simulink model "Filter_attivo"  (R2016b)
settings: Solver=ode23t  StartTime=0.0  StopTime=2.4  MaxStep=1e-4  RelTol=1e-3  EnableMultiTasking=on
values from neighbouring files (symbols this model uses):
  ampiezza_rete = 150/sqrt(3)    [Data.m]    (also in taratura.m)
  C = 2.2e-3    (= 0.0022)    [Data.m]
  C_raddr = 600e-6    (= 0.0006)    [Data.m]
  f = 50    [Data.m]    (also in Spettro_complesso.m = bar(-fp((26:25:25000-25)),PyTHD(length(PyTHD)-1:-1:length(Py)
  f_am = 500    [Data.m]
  h = Lagrange_coef(f,1/Tc)    [Data.m]    (also in Lagrange_coef.m = NaN(4,round(fc/f1*0.5)))
  h_rit = Lagrange_coef_rit(1.5)    [Data.m]
  k_interno = 0.99    [tuning.m]
  k_par_AM = 10    [Data.m]
  ki_PI = 0.2    [Data.m]
  ki_PLL = 1000    [Data.m]
  ki_ris = 47.5*2    (= 95)    [Data.m]
  kp_PI = 1.57    [Data.m]
  kp_PLL = 0.9    [Data.m]
  kp_ris = 47.5*0.089*2    (= 8.455)    [Data.m]
  L_disaccoppiamento = 2*1.18e-3    (= 0.00236)    [Data.m]    (also in taratura.m)
  L_rete = 4e-3    (= 0.004)    [Data.m]    (also in tuning.m)
  max_PI = 8    [Data.m]
  max_PLL = 1000    [Data.m]
  min_PI = -8    [Data.m]
  min_PLL = -1000    [Data.m]
  Notch_z = 1-Peaking_z    [Data.m]
  Notch_z_AM1 = 1-Peaking_z_AM1    [Notch.m]
  peak_rete = Peaking(f,1/Tc,0.1)    [Data.m]
  Peaking_dir1_d = c2d(Peaking_dir1_s,1/fs,'tustin')    [semipeaking.m]
  pendenza = 1000    [Data.m]
  R_carico = 50    [Data.m]
  R_disaccoppiamento = 2*13e-3    (= 0.026)    [Data.m]    (also in taratura.m)
  R_raddr = 60    [Data.m]
  R_rete = 100e-3    (= 0.1)    [Data.m]    (also in tuning.m = 0.01)
  T = 20e-3    (= 0.02)    [Data.m]    (also in tuning.m)
  tau_filtro_Vdc_ref = 0.15    [Data.m]
  Tc = 1/10000    (= 0.0001)    [Data.m]    (also in taratura.m; tuning.m)
  Vdc_ref = 200    [Data.m]    (also in taratura.m)
  w_filtro = 2*pi*f_taglio    (= 56548.6677646)    [Data.m]
undefined symbols (not defined in the file or in its folder): DiscIntNeverNeededParam, k_par, k_ser, Notch_z_AM1_5, Notch_z_AM1_7, Notch_z_AM2_5, Notch_z_AM2_7, Peaking_inv_d, plecs, Q_inv
libraries: powerlib x54, simulink x8, powerlib_extras x4, powerlib_meascontrol x2
(part 5 of 5)

== system Filter_attivo/Controllo tensione/Controllo ripetitivo/Controllo ripetitivo/Regolatore ripetitivo/vecchi controlli/Ripetitivo Modulazione AM1/Banco di ripetitivi/rep_comp 5 ==
  In1 : Inport
  Add1 : Sum  Inputs=-+
  Delay1 : Delay
  Delay3 : Delay  DelayLength=fix(1/(Tc*f*1*ro)-1-rit)
  Discrete FIR Filter : DiscreteFir  Coefficients=[h(1,ro) h(2,ro) h(3,ro) h(4,ro)]
  Gain : Gain  Gain=0.98
  Gain1 : Gain  Gain=g_interno
  Scope2 : Subsystem  LoadFcn=plecs('sl', 300);  InitFcn=plecs('sl', 314);  StartFcn=plecs('sl', 308);  StopFcn=plecs('sl', 309);  mask{Settings=<binary blob, 216 chars, not shown>}
      mask init:
      | plecs('sl', 315);
      settings: CopyFcn=plecs('sl', 303);  DeleteFcn=plecs('sl', 305);  UndoDeleteFcn=plecs('sl', 306);  PreSaveFcn=plecs('sl', 311);  NameChangeFcn=plecs('sl', 310);  DestroyFcn=plecs('sl', 307);  OpenFcn=plecs('sl', 302);  ErrorFcn=plerrorfcn
      mask Display: plot([0.1 0.9 0.9 0.1 0.1], [0.9 0.9 0.5 0.5 0.9])
  Out1 : Outport
  wires:
  Gain1/1 -> Out1/1, Scope2/1(1)
  Discrete FIR Filter/1 -> Gain/1, Gain1/1
  Gain/1 -> Delay1/1
  Delay1/1 -> Add1/2
  Add1/1 -> Delay3/1
  In1/1 -> Add1/1
  Delay3/1 -> Discrete FIR Filter/1

== system Filter_attivo/Controllo tensione/Controllo ripetitivo/Controllo ripetitivo/Regolatore ripetitivo/vecchi controlli/Ripetitivo Modulazione AM1/Banco di ripetitivi/rep_comp 6 ==
  In1 : Inport
  Add1 : Sum  Inputs=-+
  Delay1 : Delay
  Delay3 : Delay  DelayLength=fix(1/(Tc*f*1*ro)-1-rit)
  Discrete FIR Filter : DiscreteFir  Coefficients=[h(1,ro) h(2,ro) h(3,ro) h(4,ro)]
  Gain : Gain  Gain=0.98
  Gain1 : Gain  Gain=g_interno
  Scope2 : Subsystem  LoadFcn=plecs('sl', 300);  InitFcn=plecs('sl', 314);  StartFcn=plecs('sl', 308);  StopFcn=plecs('sl', 309);  mask{Settings=<binary blob, 216 chars, not shown>}
      mask init:
      | plecs('sl', 315);
      settings: CopyFcn=plecs('sl', 303);  DeleteFcn=plecs('sl', 305);  UndoDeleteFcn=plecs('sl', 306);  PreSaveFcn=plecs('sl', 311);  NameChangeFcn=plecs('sl', 310);  DestroyFcn=plecs('sl', 307);  OpenFcn=plecs('sl', 302);  ErrorFcn=plerrorfcn
      mask Display: plot([0.1 0.9 0.9 0.1 0.1], [0.9 0.9 0.5 0.5 0.9])
  Out1 : Outport
  wires:
  Delay3/1 -> Discrete FIR Filter/1
  In1/1 -> Add1/1
  Add1/1 -> Delay3/1
  Delay1/1 -> Add1/2
  Gain/1 -> Delay1/1
  Discrete FIR Filter/1 -> Gain1/1, Gain/1
  Gain1/1 -> Scope2/1(1), Out1/1

== system Filter_attivo/Controllo tensione/Controllo ripetitivo/Controllo ripetitivo/Regolatore ripetitivo/vecchi controlli/Ripetitivo Modulazione AM1/Banco notch 5_7_AM/notch_demodulazione_5_1 ==
  In1 : Inport
  Discrete Transfer Fcn : DiscreteTransferFcn  Numerator=cell2mat(Notch_z_AM1_5.num)  Denominator=cell2mat(Notch_z_AM1_5.den)
  Discrete Transfer Fcn1 : DiscreteTransferFcn  Numerator=cell2mat(Notch_z_AM2_5.num)  Denominator=cell2mat(Notch_z_AM2_5.den)
  Discrete Transfer Fcn2 : DiscreteTransferFcn  Numerator=cell2mat(Notch_z_AM1_7.num)  Denominator=cell2mat(Notch_z_AM1_7.den)
  Discrete Transfer Fcn3 : DiscreteTransferFcn  Numerator=cell2mat(Notch_z_AM2_7.num)  Denominator=cell2mat(Notch_z_AM2_7.den)
  Out1 : Outport
  wires:
  Discrete Transfer Fcn2/1 -> Out1/1
  In1/1 -> Discrete Transfer Fcn/1
  Discrete Transfer Fcn/1 -> Discrete Transfer Fcn1/1
  Discrete Transfer Fcn1/1 -> Discrete Transfer Fcn3/1
  Discrete Transfer Fcn3/1 -> Discrete Transfer Fcn2/1

== system Filter_attivo/Controllo tensione/Controllo ripetitivo/Controllo ripetitivo/Regolatore ripetitivo/vecchi controlli/Ripetitivo Modulazione AM1/Banco notch 5_7_AM/notch_demodulazione_5_7 ==
  In1 : Inport
  Discrete Transfer Fcn : DiscreteTransferFcn  Numerator=cell2mat(Notch_z_AM1_5.num)  Denominator=cell2mat(Notch_z_AM1_5.den)
  Discrete Transfer Fcn1 : DiscreteTransferFcn  Numerator=cell2mat(Notch_z_AM2_5.num)  Denominator=cell2mat(Notch_z_AM2_5.den)
  Discrete Transfer Fcn2 : DiscreteTransferFcn  Numerator=cell2mat(Notch_z_AM1_7.num)  Denominator=cell2mat(Notch_z_AM1_7.den)
  Discrete Transfer Fcn3 : DiscreteTransferFcn  Numerator=cell2mat(Notch_z_AM2_7.num)  Denominator=cell2mat(Notch_z_AM2_7.den)
  Out1 : Outport
  wires:
  Discrete Transfer Fcn3/1 -> Discrete Transfer Fcn2/1
  Discrete Transfer Fcn1/1 -> Discrete Transfer Fcn3/1
  Discrete Transfer Fcn/1 -> Discrete Transfer Fcn1/1
  In1/1 -> Discrete Transfer Fcn/1
  Discrete Transfer Fcn2/1 -> Out1/1

== system Filter_attivo/Controllo tensione/Controllo ripetitivo/Controllo ripetitivo/Regolatore ripetitivo/vecchi controlli/Ripetitivo Modulazione AM1/Scope1/ InputMux  ==
  In1 : Inport
  Convert1 : DataTypeConversion  SaturateOnIntegerOverflow=on  RndMeth=Zero
  Mux : Mux  Inputs=1
  Out : Outport
  wires:
  Mux/1 -> Out/1
  In1/1 -> Convert1/1
  Convert1/1 -> Mux/1

== system Filter_attivo/Controllo tensione/Controllo ripetitivo/Controllo ripetitivo/Regolatore ripetitivo/Ripetitivo Modulazione AM/Banco di ripetitivi/rep_comp 1/Scope2/ InputMux  ==
  In1 : Inport
  Convert1 : DataTypeConversion  SaturateOnIntegerOverflow=on  RndMeth=Zero
  Mux : Mux  Inputs=1
  Out : Outport
  wires:
  Mux/1 -> Out/1
  In1/1 -> Convert1/1
  Convert1/1 -> Mux/1

== system Filter_attivo/Controllo tensione/Controllo ripetitivo/Controllo ripetitivo/Regolatore ripetitivo/Ripetitivo Modulazione AM/Banco di ripetitivi/rep_comp 2/Scope2/ InputMux  ==
  In1 : Inport
  Convert1 : DataTypeConversion  SaturateOnIntegerOverflow=on  RndMeth=Zero
  Mux : Mux  Inputs=1
  Out : Outport
  wires:
  Convert1/1 -> Mux/1
  In1/1 -> Convert1/1
  Mux/1 -> Out/1

== system Filter_attivo/Controllo tensione/Controllo ripetitivo/Controllo ripetitivo/Regolatore ripetitivo/Ripetitivo Modulazione AM/Banco di ripetitivi/rep_comp 3/Scope2/ InputMux  ==
  In1 : Inport
  Convert1 : DataTypeConversion  SaturateOnIntegerOverflow=on  RndMeth=Zero
  Mux : Mux  Inputs=1
  Out : Outport
  wires:
  Mux/1 -> Out/1
  In1/1 -> Convert1/1
  Convert1/1 -> Mux/1

== system Filter_attivo/Controllo tensione/Controllo ripetitivo/Controllo ripetitivo/Regolatore ripetitivo/Ripetitivo Modulazione AM/Banco di ripetitivi/rep_comp 4/Scope2/ InputMux  ==
  In1 : Inport
  Convert1 : DataTypeConversion  SaturateOnIntegerOverflow=on  RndMeth=Zero
  Mux : Mux  Inputs=1
  Out : Outport
  wires:
  Convert1/1 -> Mux/1
  In1/1 -> Convert1/1
  Mux/1 -> Out/1

== system Filter_attivo/Controllo tensione/Controllo ripetitivo/Controllo ripetitivo/Regolatore ripetitivo/Ripetitivo Modulazione AM/Banco di ripetitivi/rep_comp 5/Scope2/ InputMux  ==
  In1 : Inport
  Convert1 : DataTypeConversion  SaturateOnIntegerOverflow=on  RndMeth=Zero
  Mux : Mux  Inputs=1
  Out : Outport
  wires:
  Mux/1 -> Out/1
  In1/1 -> Convert1/1
  Convert1/1 -> Mux/1

== system Filter_attivo/Controllo tensione/Controllo ripetitivo/Controllo ripetitivo/Regolatore ripetitivo/Ripetitivo Modulazione AM/Banco di ripetitivi/rep_comp 6/Scope2/ InputMux  ==
  In1 : Inport
  Convert1 : DataTypeConversion  SaturateOnIntegerOverflow=on  RndMeth=Zero
  Mux : Mux  Inputs=1
  Out : Outport
  wires:
  Convert1/1 -> Mux/1
  In1/1 -> Convert1/1
  Mux/1 -> Out/1

== system Filter_attivo/Controllo tensione/Controllo ripetitivo/Controllo ripetitivo/Regolatore ripetitivo/vecchi controlli/Ripetitivo Modulazione AM1/Banco di ripetitivi/rep_comp 1/Scope2 ==
  1 : Inport
  " InputMux " : Subsystem
      mask Display: disp('Mux')
  " S-Function " : S-Function  FunctionName=plecs  SFunctionDeploymentMode=off  EnableBusSupport=off
  wires:
  1/1 -> " InputMux "/1(In1)
  " InputMux "/1(Out) -> " S-Function "/1

== system Filter_attivo/Controllo tensione/Controllo ripetitivo/Controllo ripetitivo/Regolatore ripetitivo/vecchi controlli/Ripetitivo Modulazione AM1/Banco di ripetitivi/rep_comp 2/Scope2 ==
  1 : Inport
  " InputMux " : Subsystem
      mask Display: disp('Mux')
  " S-Function " : S-Function  FunctionName=plecs  SFunctionDeploymentMode=off  EnableBusSupport=off
  wires:
  " InputMux "/1(Out) -> " S-Function "/1
  1/1 -> " InputMux "/1(In1)

== system Filter_attivo/Controllo tensione/Controllo ripetitivo/Controllo ripetitivo/Regolatore ripetitivo/vecchi controlli/Ripetitivo Modulazione AM1/Banco di ripetitivi/rep_comp 3/Scope2 ==
  1 : Inport
  " InputMux " : Subsystem
      mask Display: disp('Mux')
  " S-Function " : S-Function  FunctionName=plecs  SFunctionDeploymentMode=off  EnableBusSupport=off
  wires:
  1/1 -> " InputMux "/1(In1)
  " InputMux "/1(Out) -> " S-Function "/1

== system Filter_attivo/Controllo tensione/Controllo ripetitivo/Controllo ripetitivo/Regolatore ripetitivo/vecchi controlli/Ripetitivo Modulazione AM1/Banco di ripetitivi/rep_comp 4/Scope2 ==
  1 : Inport
  " InputMux " : Subsystem
      mask Display: disp('Mux')
  " S-Function " : S-Function  FunctionName=plecs  SFunctionDeploymentMode=off  EnableBusSupport=off
  wires:
  " InputMux "/1(Out) -> " S-Function "/1
  1/1 -> " InputMux "/1(In1)

== system Filter_attivo/Controllo tensione/Controllo ripetitivo/Controllo ripetitivo/Regolatore ripetitivo/vecchi controlli/Ripetitivo Modulazione AM1/Banco di ripetitivi/rep_comp 5/Scope2 ==
  1 : Inport
  " InputMux " : Subsystem
      mask Display: disp('Mux')
  " S-Function " : S-Function  FunctionName=plecs  SFunctionDeploymentMode=off  EnableBusSupport=off
  wires:
  1/1 -> " InputMux "/1(In1)
  " InputMux "/1(Out) -> " S-Function "/1

== system Filter_attivo/Controllo tensione/Controllo ripetitivo/Controllo ripetitivo/Regolatore ripetitivo/vecchi controlli/Ripetitivo Modulazione AM1/Banco di ripetitivi/rep_comp 6/Scope2 ==
  1 : Inport
  " InputMux " : Subsystem
      mask Display: disp('Mux')
  " S-Function " : S-Function  FunctionName=plecs  SFunctionDeploymentMode=off  EnableBusSupport=off
  wires:
  " InputMux "/1(Out) -> " S-Function "/1
  1/1 -> " InputMux "/1(In1)

== system Filter_attivo/Controllo tensione/Controllo ripetitivo/Controllo ripetitivo/Regolatore ripetitivo/vecchi controlli/Ripetitivo Modulazione AM1/Banco di ripetitivi/rep_comp 1/Scope2/ InputMux  ==
  In1 : Inport
  Convert1 : DataTypeConversion  SaturateOnIntegerOverflow=on  RndMeth=Zero
  Mux : Mux  Inputs=1
  Out : Outport
  wires:
  Convert1/1 -> Mux/1
  In1/1 -> Convert1/1
  Mux/1 -> Out/1

== system Filter_attivo/Controllo tensione/Controllo ripetitivo/Controllo ripetitivo/Regolatore ripetitivo/vecchi controlli/Ripetitivo Modulazione AM1/Banco di ripetitivi/rep_comp 2/Scope2/ InputMux  ==
  In1 : Inport
  Convert1 : DataTypeConversion  SaturateOnIntegerOverflow=on  RndMeth=Zero
  Mux : Mux  Inputs=1
  Out : Outport
  wires:
  Mux/1 -> Out/1
  In1/1 -> Convert1/1
  Convert1/1 -> Mux/1

== system Filter_attivo/Controllo tensione/Controllo ripetitivo/Controllo ripetitivo/Regolatore ripetitivo/vecchi controlli/Ripetitivo Modulazione AM1/Banco di ripetitivi/rep_comp 3/Scope2/ InputMux  ==
  In1 : Inport
  Convert1 : DataTypeConversion  SaturateOnIntegerOverflow=on  RndMeth=Zero
  Mux : Mux  Inputs=1
  Out : Outport
  wires:
  Convert1/1 -> Mux/1
  In1/1 -> Convert1/1
  Mux/1 -> Out/1

== system Filter_attivo/Controllo tensione/Controllo ripetitivo/Controllo ripetitivo/Regolatore ripetitivo/vecchi controlli/Ripetitivo Modulazione AM1/Banco di ripetitivi/rep_comp 4/Scope2/ InputMux  ==
  In1 : Inport
  Convert1 : DataTypeConversion  SaturateOnIntegerOverflow=on  RndMeth=Zero
  Mux : Mux  Inputs=1
  Out : Outport
  wires:
  Mux/1 -> Out/1
  In1/1 -> Convert1/1
  Convert1/1 -> Mux/1

== system Filter_attivo/Controllo tensione/Controllo ripetitivo/Controllo ripetitivo/Regolatore ripetitivo/vecchi controlli/Ripetitivo Modulazione AM1/Banco di ripetitivi/rep_comp 5/Scope2/ InputMux  ==
  In1 : Inport
  Convert1 : DataTypeConversion  SaturateOnIntegerOverflow=on  RndMeth=Zero
  Mux : Mux  Inputs=1
  Out : Outport
  wires:
  Convert1/1 -> Mux/1
  In1/1 -> Convert1/1
  Mux/1 -> Out/1

== system Filter_attivo/Controllo tensione/Controllo ripetitivo/Controllo ripetitivo/Regolatore ripetitivo/vecchi controlli/Ripetitivo Modulazione AM1/Banco di ripetitivi/rep_comp 6/Scope2/ InputMux  ==
  In1 : Inport
  Convert1 : DataTypeConversion  SaturateOnIntegerOverflow=on  RndMeth=Zero
  Mux : Mux  Inputs=1
  Out : Outport
  wires:
  Mux/1 -> Out/1
  In1/1 -> Convert1/1
  Convert1/1 -> Mux/1

== matlab function Filter_attivo/Rete/generatore diretta e inversa/MATLAB Function ==
  data: teta input; v_a output; a_d input; a_i input; v_b output; v_c output; fase_i input
function [v_a,v_b,v_c] = fcn(teta,a_d,a_i,fase_i)

alfa=exp(2/3*pi*1i);
alfa_q=exp(-2/3*pi*1i);
vd_c=a_d*exp(-teta*1i);
v1_d=real(vd_c);
v2_d=real(vd_c*alfa_q);
v3_d=real(vd_c*alfa);
vi_c=a_i*exp((teta-fase_i)*1i);
v1_i=real(vi_c);
v2_i=real(vi_c*alfa_q);
v3_i=real(vi_c*alfa);
v_a=v1_i+v1_d;
v_b=v2_i+v2_d;
v_c=v3_i+v3_d;
% v_c=-v_a-v_b;

== matlab function Filter_attivo/Controllo tensione/Controllo PR 10 kHz/controllo bus DC/PI antiwindup/Embedded MATLAB Function ==
  data: error input; out output; kp input; ki input; min input; max input; Tc parameter
function out = fcn(error,kp,ki,min,max,Tc)
% Regolator PI con antiwindup.
% Discretizzazione con Eulero all'indietro.

persistent start
persistent error_p
persistent out_p

if (isempty(start))
    start=1;
    error_p=0;
    out_p=0;
end

out=out_p+kp*(error-error_p)+ki*error*Tc;

if out>max
    out=max;
    error=(max-out_p+(kp*error_p))/(kp+(ki*Tc));
elseif out<min
    out=min;
    error=(min-out_p+(kp*error_p))/(kp+(ki*Tc));
end

out_p=out;
error_p=error;

== matlab function Filter_attivo/Controllo tensione/Controllo PR 10 kHz/controllo bus DC/PI antiwindup1/Embedded MATLAB Function ==
  data: error input; out output; kp input; ki input; min input; max input; Tc parameter
function out = fcn(error,kp,ki,min,max,Tc)
% Regolator PI con antiwindup.
% Discretizzazione con Eulero all'indietro.

persistent start
persistent error_p
persistent out_p

if (isempty(start))
    start=1;
    error_p=0;
    out_p=0;
end

out=out_p+kp*(error-error_p)+ki*error*Tc;

if out>max
    out=max;
    error=(max-out_p+(kp*error_p))/(kp+(ki*Tc));
elseif out<min
    out=min;
    error=(min-out_p+(kp*error_p))/(kp+(ki*Tc));
end

out_p=out;
error_p=error;

== matlab function Filter_attivo/Controllo tensione/Controllo PR 10 kHz/controllo bus DC/Filtro passa-basso tempo discreto/Embedded MATLAB Function ==
  data: in input; out output; tau input; Tc parameter; Vdc input; avvio input
function out = fcn(in,tau,Tc,Vdc,avvio)
% Filtro passa-basso tempo discreto.
% Discretizzazione con Eulero all'indietro.

persistent start
persistent out_p

if (isempty(start))
    start=1;
    out_p=0;  
end

if (avvio==0)
    out=Vdc;   
else

out=(tau/(tau+Tc))*out_p+(Tc/(tau+Tc))*(in);
end
out_p=out;

== matlab function Filter_attivo/Controllo tensione/Controllo PR 10 kHz/PLL_tempo_discreto/PI antiwindup/Embedded MATLAB Function ==
  data: error input; out output; kp input; ki input; min input; max input; Tc parameter
function out = fcn(error,kp,ki,min,max,Tc)
% Regolatore PI con antiwindup.
% Discretizzazione con Eulero all'indietro.

persistent start
persistent error_p
persistent out_p

if (isempty(start))
    start=1;
    error_p=0;
    out_p=0;
end

out=out_p+kp*(error-error_p)+ki*error*Tc;

if out>max
    out=max;
    error=(max-out_p+(kp*error_p))/(kp+(ki*Tc));
elseif out<min
    out=min;
    error=(min-out_p+(kp*error_p))/(kp+(ki*Tc));
end

out_p=out;
error_p=error;

== matlab function Filter_attivo/Controllo tensione/Controllo PR 10 kHz/Controllo risonante/Contributo controllo risonante fondamentale/PIR_tustin_prewarp/MATLAB Function ==
  data: error input; out output; kp input; ki input; min input; max input; Tc input; delta input; w0 input
function out = fcn(error,kp,ki,min,max,Tc,delta,w0)
% Regolator PIR con antiwindup.
% Discretizzazione con Eulero all'indietro con prewarp.

persistent start
persistent error_p
persistent error_pp
persistent out_p
persistent out_pp

if (isempty(start))
    start=1;
    error_p=0;
    out_p=0;
    error_pp=0;
    out_pp=0;
end

k1=1/(1-delta*sin(w0*Tc));
k2=1+delta*sin(w0*Tc);
k3=ki/2/w0;

out=kp*error+k1*(2*cos(w0*Tc)*(out_p-kp*error_p)-k2*(out_pp-kp*error_pp)-k3*(error+2*error_p+error_pp));

k=k1*(2*cos(w0*Tc)*(out_p-kp*error_p)-k2*(out_pp-kp*error_pp)-k3*(2*error_p+error_pp));

if out>max
    out=max;
    error=(max-k)/(kp+k3*k1);
elseif out<min
    out=min;
    error=(min-k)/(kp+k3*k1);
end

out_pp=out_p;
out_p=out;
error_pp=error_p;
error_p=error;

== matlab function Filter_attivo/Controllo tensione/Controllo PR 10 kHz/Controllo risonante/Contributo controllo risonante fondamentale/PIR_tustin_prewarp/MATLAB Function1 ==
  data: error input; out output; kp input; ki input; min input; max input; Tc input; delta input; w0 input
function out = fcn(error,kp,ki,min,max,Tc,delta,w0)
% Regolator PIR con antiwindup.
% Discretizzazione con Eulero all'indietro con prewarp.

persistent start
persistent error_p
persistent error_pp
persistent out_p
persistent out_pp

if (isempty(start))
    start=1;
    error_p=0;
    out_p=0;
    error_pp=0;
    out_pp=0;
end

k1=1/(1-delta*sin(w0*Tc));
k2=1+delta*sin(w0*Tc);
k3=ki/2/w0;

out=kp*error+k1*(2*cos(w0*Tc)*(out_p-kp*error_p)-k2*(out_pp-kp*error_pp)-k3*(error+2*error_p+error_pp));

k=k1*(2*cos(w0*Tc)*(out_p-kp*error_p)-k2*(out_pp-kp*error_pp)-k3*(2*error_p+error_pp));

if out>max
    out=max;
    error=(max-k)/(kp+k3*k1);
elseif out<min
    out=min;
    error=(min-k)/(kp+k3*k1);
end

out_pp=out_p;
out_p=out;
error_pp=error_p;
error_p=error;

== matlab function Filter_attivo/Controllo tensione/Controllo ripetitivo/Controllo ripetitivo con downsampling/Regolatore ripetitivo/ buffer intero fase zero-riduzione di 1/Embedded MATLAB Function1 ==
  data: error input; out output; n input
function out = fcn(error,n)
% filtro FIR per arrotondamento

persistent start
persistent error_p
persistent error_pp
persistent error_ppp

f1=50;
f1c=10000;

if (isempty(start))
    start=1;
    error_p=0;
    error_pp=0;
    error_ppp=0;
    
end

if ((f1c/f1/n)-fix(f1c/f1/n)) == 0
    out=error_p;
    
else
    
    h=zeros(1,4);
    D=(f1c/f1/n)-(fix(f1c/f1/n)-1); %delay da approssimare
    
    h(1)=-(D-1)*(D-2)*(D-3)/6;
    h(2)=D*(D-2)*(D-3)/2;
    h(3)=-D*(D-1)*(D-3)/2;
    h(4)=D*(D-1)*(D-2)/6;
    
    out= h(1)*error+h(2)*error_p+h(3)*error_pp+h(4)*error_ppp;
    
    error_p=error;
    error_pp=error_p;
    error_ppp=error_pp;
end
end

== matlab function Filter_attivo/Controllo tensione/Controllo PR 10 kHz/controllo /PI antiwindup/Embedded MATLAB Function ==
  data: error input; out output; kp input; ki input; min input; max input; Tc parameter
function out = fcn(error,kp,ki,min,max,Tc)
% Regolator PI con antiwindup.
% Discretizzazione con Eulero all'indietro.

persistent start
persistent error_p
persistent out_p

if (isempty(start))
    start=1;
    error_p=0;
    out_p=0;
end

out=out_p+kp*(error-error_p)+ki*error*Tc;

if out>max
    out=max;
    error=(max-out_p+(kp*error_p))/(kp+(ki*Tc));
elseif out<min
    out=min;
    error=(min-out_p+(kp*error_p))/(kp+(ki*Tc));
end

out_p=out;
error_p=error;

== matlab function Filter_attivo/Controllo tensione/Controllo ripetitivo/Controllo ripetitivo con downsampling/Regolatore ripetitivo/ buffer intero fase zero-riduzione di 1/Embedded MATLAB Function2 ==
  data: error input; out output; n input
function out = fcn(error,n)
% filtro FIR per arrotondamento

persistent start
persistent error_p
persistent error_pp
persistent error_ppp

f1=50;
f1c=10000;

if (isempty(start))
    start=1;
    error_p=0;
    error_pp=0;
    error_ppp=0;
    
end

if ((f1c/f1/n)-fix(f1c/f1/n)) == 0
    out=error_p;
    
else
    h=zeros(1,4);
    D=(f1c/f1/n)-(fix(f1c/f1/n)-1); %delay da approssimare
    
    h(1)=-(D-1)*(D-2)*(D-3)/6;
    h(2)=D*(D-2)*(D-3)/2;
    h(3)=-D*(D-1)*(D-3)/2;
    h(4)=D*(D-1)*(D-2)/6;
    
    out= h(1)*error+h(2)*error_p+h(3)*error_pp+h(4)*error_ppp;
    
    error_p=error;
    error_pp=error_p;
    error_ppp=error_pp;
end
end

== matlab function Filter_attivo/Controllo tensione/Controllo ripetitivo/Controllo ripetitivo con downsampling/Regolatore ripetitivo/ buffer metà fase zero/k_serie step/MATLAB Function ==
  data: k output; Tc input; k_partenza input; step_t input; step_y input
function k  = fcn(Tc,k_partenza,step_t,step_y)

persistent y_p;
persistent count;

if isempty(y_p)
    y_p=k_partenza;
    count=0;
end
count=count+1;
if (count>=round(step_t/Tc))
    k=y_p+step_y;
    y_p=k;
    count=0;
else
    k=y_p;
end

== matlab function Filter_attivo/Controllo tensione/Controllo ripetitivo/Controllo ripetitivo con downsampling/Regolatore ripetitivo/ buffer metà fase zero-riduzione di 3/k_serie step/MATLAB Function ==
  data: k output; Tc input; k_partenza input; step_t input; step_y input
function k  = fcn(Tc,k_partenza,step_t,step_y)

persistent y_p;
persistent count;

if isempty(y_p)
    y_p=k_partenza;
    count=0;
end
count=count+1;
if (count>=round(step_t/Tc))
    k=y_p+step_y;
    y_p=k;
    count=0;
else
    k=y_p;
end

== matlab function Filter_attivo/Controllo tensione/Controllo ripetitivo/Controllo ripetitivo con downsampling/Regolatore ripetitivo/ buffer metà mattavelli/k_serie step/MATLAB Function ==
  data: k output; Tc input; k_partenza input; step_t input; step_y input
function k  = fcn(Tc,k_partenza,step_t,step_y)

persistent y_p;
persistent count;

if isempty(y_p)
    y_p=k_partenza;
    count=0;
end
count=count+1;
if (count>=round(step_t/Tc))
    k=y_p+step_y;
    y_p=k;
    count=0;
else
    k=y_p;
end

== matlab function Filter_attivo/Controllo tensione/Controllo ripetitivo/Controllo ripetitivo/Regolatore ripetitivo/vecchi controlli/Generatore step /MATLAB Function ==
  data: y output; Tc input; k_partenza input; step_t input; step_y input
function y  = fcn(Tc,k_partenza,step_t,step_y)

persistent y_p;
persistent count;

if isempty(y_p)
    y_p=k_partenza;
    count=0;
end
count=count+1;
if (count>=round(step_t/Tc))
    y=y_p+step_y;
    y_p=y;
    count=0;
else
    y=y_p;
end

== matlab function Filter_attivo/Controllo tensione/Controllo ripetitivo/Controllo ripetitivo/Regolatore ripetitivo/vecchi controlli/ Ripetitivo buffer intero/k_serie step/MATLAB Function ==
  data: k output; Tc input; k_partenza input; step_t input; step_y input
function k  = fcn(Tc,k_partenza,step_t,step_y)

persistent y_p;
persistent count;

if isempty(y_p)
    y_p=k_partenza;
    count=0;
end
count=count+1;
if (count>=round(step_t/Tc))
    k=y_p+step_y;
    y_p=k;
    count=0;
else
    k=y_p;
end

== matlab function Filter_attivo/Controllo tensione/Controllo ripetitivo/Controllo ripetitivo/Regolatore ripetitivo/vecchi controlli/ Ripetitivo buffer intero1.5 di ritardo/k_serie step/MATLAB Function ==
  data: k output; Tc input; k_partenza input; step_t input; step_y input
function k  = fcn(Tc,k_partenza,step_t,step_y)

persistent y_p;
persistent count;

if isempty(y_p)
    y_p=k_partenza;
    count=0;
end
count=count+1;
if (count>=round(step_t/Tc))
    k=y_p+step_y;
    y_p=k;
    count=0;
else
    k=y_p;
end

== matlab function Filter_attivo/Controllo tensione/Controllo ripetitivo/Controllo ripetitivo/Regolatore ripetitivo/vecchi controlli/ buffer intero mattavelli buchi amplificati/k_serie step/MATLAB Function ==
  data: k output; Tc input; k_partenza input; step_t input; step_y input
function k  = fcn(Tc,k_partenza,step_t,step_y)

persistent y_p;
persistent count;

if isempty(y_p)
    y_p=k_partenza;
    count=0;
end
count=count+1;
if (count>=round(step_t/Tc))
    k=y_p+step_y;
    y_p=k;
    count=0;
else
    k=y_p;
end
